simulink model "dbx_control"  (R2015a)
settings: Solver=FixedStepDiscrete  SolverMode=SingleTasking  StartTime=0.0  StopTime=20  FixedStep=T_ctrl  RelTol=1e-3
undefined symbols (not defined in the file): A_l_max_x, A_M, A_z_max, CG, epsilon, Flaps_ang_deg, g, Hover_eta_23, Hover_throtle_1, Hover_throtle_23, I_BAC, L_M, m, Roll_pich_sens, Servo_calib, T_ctrl, Throtle_sens, v_i0, Yaw_sens
libraries: DBX_model x29, DBX_Control_lib x15, simulink x8, DBX_Control x3
(part 2 of 2)

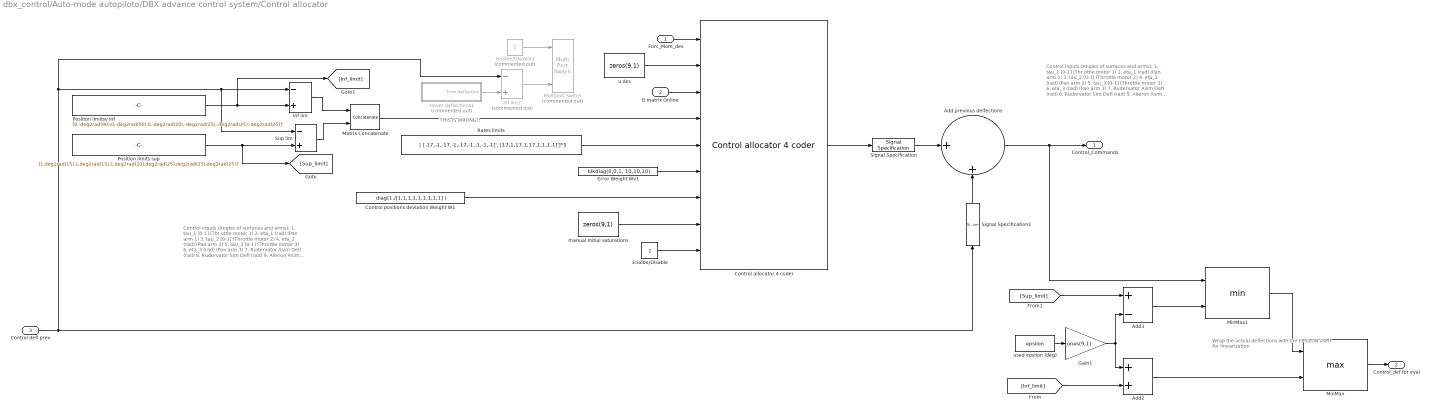
== system dbx_control/Auto-mode autopiloto/DBX advance control system/Control allocator ==
  note: THIS IS WRONG!!
  note: Wrap the actual deflections with the EPSILON
      |  used for linearization
  note: Control inputs (Angles  of surfaces and arms):
      |
      | 1. tau_1 [0-1] (Thr ottle motor 1)
      | 2. eta_1 (rad)  (Pan arm 1)
      |
      | 3. tau_2 [0-1] (Throttle motor 2)
      | 4. eta_2 (rad)  (Pan arm 2)
      |
      | 5. tau_3 [0-1] (Throttle motor 3)
      | 6. eta_3 (rad)  (Pan arm  3)
      |
      | 7. Rudervator Asim Defl (rad)
      | 8. Rudervator Sim Defl (rad)
      | 9. Aileron Asim Defl (rad)
  note: Control inputs (Angles  of surfaces and arms):
      |
      | 1. tau_1 [0-1] (Thr ottle motor 1)
      | 2. eta_1 (rad)  (Pan arm 1)
      |
      | 3. tau_2 [0-1] (Throttle motor 2)
      | 4. eta_2 (rad)  (Pan arm 2)
      |
      | 5. tau_3 [0-1] (Throttle motor 3)
      | 6. eta_3 (rad)  (Pan arm  3)
      |
      | 7. Rudervator Asim Defl (rad)
      | 8. Rudervator Sim Defl (rad)
      | 9. Aileron Asim Defl (rad)
  Forc_Mom_des : Inport
  B matrix Online : Inport  Port=2
  Control defl prev : Inport  Port=3
  Add previous delfections : Sum  Inputs=|++
  Add2 : Sum
  Add3 : Sum  Inputs=+-
  Control allocator 4 coder : DBX_Control_lib/Control allocator 4 coder  gamma=1  imax=20  T=T_ctrl
  Control positions deviation Weight W1 : Constant  Value=diag(1./[1,1,1,1,1,1,1,1,1] )
  Enalbe/Disable : Constant
  Enalbe/Disable1 : Constant  Commented=on
  Error Weight Wv1 : Constant  Value=blkdiag(0,0,1, 10,10,10)
  Gain1 : Gain  Gain=ones(9,1)
  Hover deflections1 : Subsystem  Commented=on  TreatAsAtomicUnit=on
  Inf lim : Sum  Inputs=-+
  Inf lim2 : Sum  Commented=on  Inputs=-+
  Matrix Concatenate : Concatenate  Mode=Multidimensional array  ConcatenateDimension=2
  MinMax : MinMax  Function=max  Inputs=2
  MinMax1 : MinMax  Inputs=2
  Multiport Switch : MultiPortSwitch  Commented=on  Inputs=2
  Position limits sup : Constant  Value=[1,deg2rad(15),1,deg2rad(15),1,deg2rad(20),deg2rad(25),deg2rad(25),deg2rad(25)]'
  Position limitsv inf : Constant  Value=[0,-deg2rad(90),0,-deg2rad(90),0,-deg2rad(20),-deg2rad(25),-deg2rad(25),-deg2rad(25)]'
  Rates limits : Constant  Value=[ [-17,-1,-17,-1,-17,-1,-1,-1,-1]', [17,1,17,1,17,1,1,1,1]']*5
  Signal Specification : SignalSpecification  Dimensions=[9,1]
  Signal Specification1 : SignalSpecification  Dimensions=[9,1]
  Sup lim : Sum  Inputs=-+
  manual Initial saturations : Constant  Value=zeros(9,1)
  u des : Constant  Value=zeros(9,1)
  used epsilon (deg) : Constant  Value=epsilon
  Control_Commands : Outport
  Control_def for eval : Outport  Port=2
  wires:
  MinMax1/1 -> MinMax/1
  Add3/1 -> MinMax1/2
  used epsilon (deg)/1 -> Gain1/1
  Gain1/1 -> Add3/2, Add2/1
  Add2/1 -> MinMax/2
  Control positions deviation Weight W1/1 -> Control allocator 4 coder/7
  Control allocator 4 coder/1 -> Signal Specification/1
  Enalbe/Disable/1 -> Control allocator 4 coder/9
  manual Initial saturations/1 -> Control allocator 4 coder/8
  Sup lim/1 -> Matrix Concatenate/2
  Inf lim/1 -> Matrix Concatenate/1
  Position limitsv inf/1 -> [Inf_limit], Inf lim/2
  Position limits sup/1 -> [Sup_limit], Sup lim/2
  Rates limits/1 -> Control allocator 4 coder/5
  Add previous delfections/1 -> Control_Commands/1, MinMax1/1
  B matrix Online/1 -> Control allocator 4 coder/3
  Signal Specification/1 -> Add previous delfections/1
  Signal Specification1/1 -> Add previous delfections/2
  Forc_Mom_des/1 -> Control allocator 4 coder/1
  Matrix Concatenate/1 -> Control allocator 4 coder/4
  Control defl prev/1 -> Inf lim2/1, Inf lim/1, Sup lim/1, Signal Specification1/1
  Inf lim2/1 -> Multiport Switch/3
  Hover deflections1/1(Trim deflectins) -> Inf lim2/2
  MinMax/1 -> Control_def for eval/1
  Error Weight Wv1/1 -> Control allocator 4 coder/6
  [Inf_limit] -> Add2/2
  [Sup_limit] -> Add3/1
  Enalbe/Disable1/1 -> Multiport Switch/1
  u des/1 -> Control allocator 4 coder/2

== system dbx_control/Auto-mode autopiloto/DBX advance control system/Deflex de-mixer ==
  note: Control outputs:
      |
      | 7. Rudervator Left (rad)
      | 8. Rudervator Right (rad)
      | 9. Aileron Left (rad)
      | 10. Aielron Right (rad)
  delta_rv_Asim : Inport
  delta_rv_sim : Inport  Port=2
  delta_ail_Asim : Inport  Port=3
  delta_ail_sim : Inport  Port=4
  Add : Sum  Inputs=|++
  Add1 : Sum  Inputs=|-+
  Add2 : Sum  Inputs=|++
  Add3 : Sum  Inputs=|-+
  delta_rv_L : Outport
  delta_rv_R : Outport  Port=2
  delta_a_L : Outport  Port=3
  delta_a_R : Outport  Port=4
  wires:
  delta_rv_Asim/1 -> Add1/1, Add/1
  Add/1 -> delta_rv_L/1
  delta_rv_sim/1 -> Add1/2, Add/2
  Add1/1 -> delta_rv_R/1
  delta_ail_Asim/1 -> Add3/1, Add2/1
  Add2/1 -> delta_a_L/1
  delta_ail_sim/1 -> Add2/2, Add3/2
  Add3/1 -> delta_a_R/1

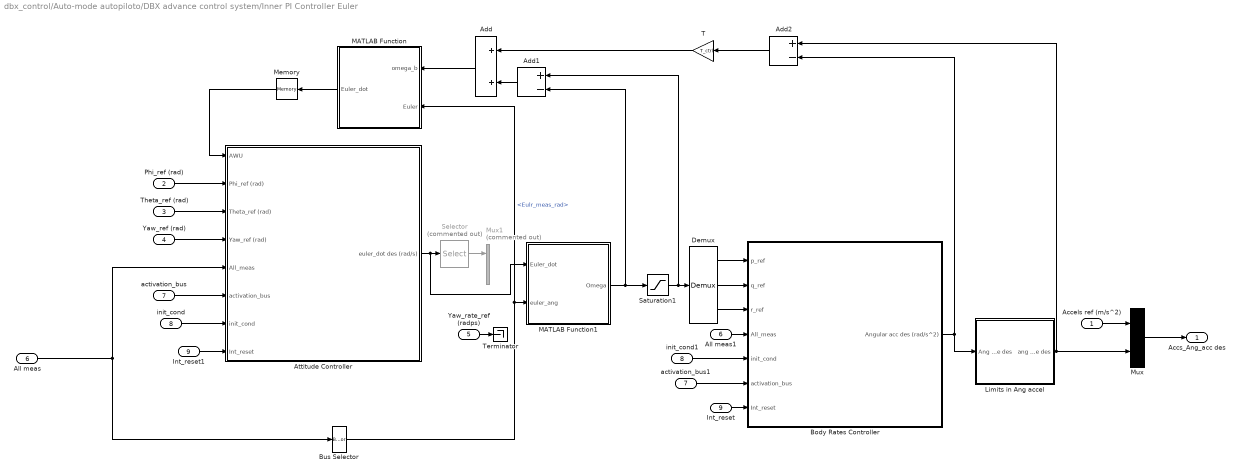
== system dbx_control/Auto-mode autopiloto/DBX advance control system/Inner PI Controller Euler ==
  Accels ref (m/s^2) : Inport
  Phi_ref (rad) : Inport  Port=2
  Theta_ref (rad) : Inport  Port=3
  Yaw_ref (rad) : Inport  Port=4
  Yaw_rate_ref (radps) : Inport  Port=5
  All meas : Inport  Port=6
  activation_bus : Inport  Port=7
  init_cond : Inport  Port=8
  Int_reset : Inport  Port=9
  Add : Sum
  Add1 : Sum  Inputs=+-
  Add2 : Sum  Inputs=+-
  All meas1 : InportShadow  Port=6
  Attitude Controller : Subsystem
  Body Rates Controller : Subsystem
  Bus Selector : BusSelector  OutputSignals=Meas.Eulr_meas_rad
  Demux : Demux  Outputs=3
  Int_reset1 : InportShadow  Port=9
  Limits in Ang accel : Subsystem  TreatAsAtomicUnit=on
  MATLAB Function : MATLAB Function  TreatAsAtomicUnit=on
  MATLAB Function1 : MATLAB Function  TreatAsAtomicUnit=on
  Memory : Memory
  Mux : Mux  Inputs=2
  Mux1 : Mux  Commented=on  Inputs=[2,1]
  Saturation1 : Saturate  UpperLimit=deg2rad(50)*[1,10,0.5]'  LowerLimit=-deg2rad(50)*[1,10,0.5]'
  Selector : Selector  Commented=on  InputPortWidth=3  Indices=[1 2]
  T : Gain  Gain=T_ctrl
  Terminator : Terminator
  activation_bus1 : InportShadow  Port=7
  init_cond1 : InportShadow  Port=8
  Accs_Ang_acc des : Outport
  wires:
  Accels ref (m/s^2)/1 -> Mux/1
  Mux/1 -> Accs_Ang_acc des/1
  All meas/1 -> Bus Selector/1, Attitude Controller/5(All_meas)
  Bus Selector/1 -> MATLAB Function/2(Euler), MATLAB Function1/2(euler_ang)  "<Eulr_meas_rad>"
  Demux/1 -> Body Rates Controller/1(p_ref)
  Demux/2 -> Body Rates Controller/2(q_ref)
  Demux/3 -> Body Rates Controller/3(r_ref)
  Phi_ref (rad)/1 -> Attitude Controller/2(Phi_ref (rad))
  Yaw_ref (rad)/1 -> Attitude Controller/4(Yaw_ref (rad))
  Limits in Ang accel/1(ang Ace des) -> Add2/1, Mux/2
  MATLAB Function1/1(Omega) -> Add1/2, Saturation1/1
  Body Rates Controller/1(Angular acc des (rad/s^2)) -> Add2/2, Limits in Ang accel/1(Ang Ace des)
  Add/1 -> MATLAB Function/1(omega_b)
  Add2/1 -> T/1
  Add1/1 -> Add/2
  T/1 -> Add/1
  MATLAB Function/1(Euler_dot) -> Memory/1
  init_cond/1 -> Attitude Controller/7(init_cond)
  activation_bus/1 -> Attitude Controller/6(activation_bus)
  All meas1/1 -> Body Rates Controller/4(All_meas)
  Saturation1/1 -> Add1/1, Demux/1
  Memory/1 -> Attitude Controller/1(AWU)
  Theta_ref (rad)/1 -> Attitude Controller/3(Theta_ref (rad))
  Selector/1 -> Mux1/1
  Attitude Controller/1(euler_dot des (rad/s)) -> MATLAB Function1/1(Euler_dot), Selector/1
  Int_reset/1 -> Body Rates Controller/7(Int_reset)
  Int_reset1/1 -> Attitude Controller/8(Int_reset)
  activation_bus1/1 -> Body Rates Controller/6(activation_bus)
  init_cond1/1 -> Body Rates Controller/5(init_cond)
  Yaw_rate_ref (radps)/1 -> Terminator/1

== system dbx_control/Auto-mode autopiloto/DBX advance control system/NDI//INDI and Grad4CA ==
  pseudo_control (m/s^2;rad/s^2) : Inport
  Control_defl for eval : Inport  Port=2
  All_meas : Inport  Port=3
  INDI and NDI : Subsystem  RTWFcnName=abc  RTWFileName=asas  VariantControl=NDI_INDI
      settings: RTWFcnNameOpts=User specified  RTWFileNameOpts=User specified
  NDI : Subsystem  RTWFcnName=abc  RTWFileName=asas  VariantControl=NDI
      settings: RTWFcnNameOpts=User specified  RTWFileNameOpts=User specified
  NDI incremental gradient : Subsystem  RTWFcnName=abc  RTWFileName=asas  VariantControl=NDI_incremental_grad
      settings: RTWFcnNameOpts=User specified  RTWFileNameOpts=User specified
  Virtual Control Commands : Outport
  B online : Outport  Port=2
  Control_defl eval (rad) : Outport  Port=3

== system dbx_control/Auto-mode autopiloto/DBX advance control system/Outter Overactuated P Controller ==
  Vel_yaw_ref(m) : Inport
  All meas : Inport  Port=2
  activation_bus : Inport  Port=3
  init_cond : Inport  Port=4
  Int_reset : Inport  Port=5
  Bus Selector1 : BusSelector  OutputSignals=Params.T_Fe_Fyaw,Meas.V_yaw,Params.DCM
  Demux2 : Demux  Outputs=3
  Matrix Multiply1 : Product  Multiplication=Matrix(*)
  Matrix Multiply3 : Product  Multiplication=Matrix(*)
  Permute Dimensions : PermuteDimensions
  Permute Dimensions1 : PermuteDimensions
  Saturation : Saturate  UpperLimit=[A_l_max_x,10,g]  LowerLimit=-[A_l_max_x,10,A_z_max-g]
  Saturation1 : Saturate  UpperLimit=[10,10,v_i0]'  LowerLimit=-[10,10,2*v_i0]'
  Terminator : Terminator
  Velocity Controller : Subsystem
  Accels des : Outport
  wires:
  Demux2/3 -> Velocity Controller/2(Vyaw_z_ref)
  Demux2/1 -> Velocity Controller/1(Vyaw_x_ref)
  All meas/1 -> Bus Selector1/1
  Bus Selector1/3 -> Permute Dimensions/1  "<DCM>"
  Matrix Multiply1/1 -> Accels des/1
  Permute Dimensions/1 -> Matrix Multiply1/1
  Saturation1/1 -> Demux2/1
  Saturation/1 -> Matrix Multiply3/2
  Bus Selector1/1 -> Permute Dimensions1/1  "<T_Fe_Fyaw>"
  Vel_yaw_ref(m)/1 -> Saturation1/1
  Matrix Multiply3/1 -> Matrix Multiply1/2  "in F_e"
  Permute Dimensions1/1 -> Matrix Multiply3/1
  Velocity Controller/1(Acc_yaw des (m/s)) -> Saturation/1
  activation_bus/1 -> Velocity Controller/4(activation_bus)
  Bus Selector1/2 -> Velocity Controller/3(V_yaw_meas)  "<V_yaw>"
  init_cond/1 -> Velocity Controller/5(Init_cond)
  Demux2/2 -> Terminator/1
  Int_reset/1 -> Velocity Controller/6(Int_reset)

== system dbx_control/Auto-mode autopiloto/DBX advance control system/keep -90//90 ==
  in (rad) : Inport
  Constant : Constant  Value=180
  Constant2 : Constant  Value=360
  Gain : Gain  Gain=360
  Math Function2 : Math  Operator=rem  SaturateOnIntegerOverflow=on
  Product : Product  Inputs=*/  RndMeth=Zero
  Rounding Function : Rounding  Operator=fix
  Sum2 : Sum  Inputs=|-+
  deg2rad1 : Gain  Gain=pi/180  SaturateOnIntegerOverflow=on  OutDataTypeStr=Inherit: Same as input  ParamDataTypeStr=Inherit: Same as input
  rad2deg : Gain  Gain=180/pi  SaturateOnIntegerOverflow=on  OutDataTypeStr=Inherit: Same as input  ParamDataTypeStr=Inherit: Same as input
  out (rad) : Outport
  wires:
  deg2rad1/1 -> out (rad)/1
  Sum2/1 -> deg2rad1/1
  Math Function2/1 -> Sum2/2, Product/1
  Constant2/1 -> Math Function2/2
  rad2deg/1 -> Math Function2/1
  Gain/1 -> Sum2/1
  Rounding Function/1 -> Gain/1
  Product/1 -> Rounding Function/1
  Constant/1 -> Product/2
  in (rad)/1 -> rad2deg/1

== system dbx_control/Auto-mode autopiloto/DBX advance control system/Control allocator/Hover deflections1 ==
  Contro Inputs1 : Constant  Value=Hover_throtle_1
  Contro Inputs2 : Constant  Value=Hover_throtle_23
  Contro Inputs3 : Constant  Value=Hover_eta_23
  Gain : Gain  Gain=-1
  Ground : Ground
  Mux : Mux  Inputs=9
  Trim deflectins : Outport
  wires:
  Contro Inputs1/1 -> Mux/1
  Contro Inputs2/1 -> Mux/7, Mux/4
  Ground/1 -> Mux/2, Mux/6, Mux/9, Mux/3
  Contro Inputs3/1 -> Gain/1, Mux/5
  Gain/1 -> Mux/8
  Mux/1 -> Trim deflectins/1

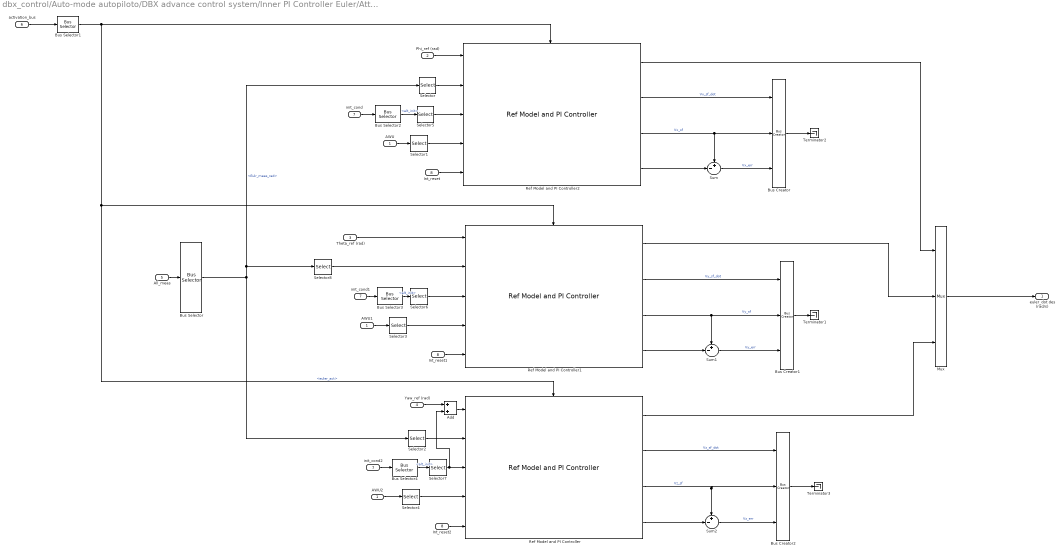
== system dbx_control/Auto-mode autopiloto/DBX advance control system/Inner PI Controller Euler/Attitude Controller ==
  AWU : Inport
  Phi_ref (rad) : Inport  Port=2
  Theta_ref (rad) : Inport  Port=3
  Yaw_ref (rad) : Inport  Port=4
  All_meas : Inport  Port=5
  activation_bus : Inport  Port=6
  init_cond : Inport  Port=7
  Int_reset : Inport  Port=8
  AWU1 : InportShadow
  AWU2 : InportShadow
  Add : Sum
  Bus Creator : BusCreator  Inputs=3
  Bus Creator1 : BusCreator  Inputs=3
  Bus Creator2 : BusCreator  Inputs=3
  Bus Selector : BusSelector  OutputSignals=Meas.Eulr_meas_rad
  Bus Selector1 : BusSelector  OutputSignals=euler_act
  Bus Selector2 : BusSelector  OutputSignals=alt_init
  Bus Selector3 : BusSelector  OutputSignals=alt_init
  Bus Selector4 : BusSelector  OutputSignals=alt_init
  Int_reset1 : InportShadow  Port=8
  Int_reset2 : InportShadow  Port=8
  Mux : Mux  Inputs=3
  Ref Model and PI Controller : DBX_Control_lib/Ref Model and PI Controller  delta=0  tau=psi_tau  RisingSlewLimit=deg2rad(20)  FallingSlewLimit=-deg2rad(20)  K_f=0  K_a=1  Con_way=pro  omega_n=4  xi=0.5  Z1=-30  K_b=psi_K_b  f_i=psi_f_i  f_c=1
  Ref Model and PI Controller1 : DBX_Control_lib/Ref Model and PI Controller  delta=0  tau=theta_tau  RisingSlewLimit=deg2rad(20)  FallingSlewLimit=-deg2rad(20)  K_f=0  K_a=1  Con_way=pro  omega_n=4  xi=0.5  Z1=-30  K_b=theta_K_b  f_i=theta_f_i  f_c=1
  Ref Model and PI Controller2 : DBX_Control_lib/Ref Model and PI Controller  delta=0  tau=phi_tau  RisingSlewLimit=deg2rad(20)  FallingSlewLimit=-deg2rad(20)  K_f=0  K_a=1  Con_way=pro  omega_n=4  xi=0.5  Z1=-30  K_b=phi_K_b  f_i=phi_f_i  f_c=1
  Selector : Selector  InputPortWidth=3
  Selector1 : Selector  InputPortWidth=3
  Selector2 : Selector  InputPortWidth=3  Indices=3
  Selector3 : Selector  InputPortWidth=3  Indices=2
  Selector4 : Selector  InputPortWidth=3  Indices=3
  Selector5 : Selector  InputPortWidth=3
  Selector6 : Selector  InputPortWidth=3  Indices=2
  Selector7 : Selector  InputPortWidth=3  Indices=3
  Selector8 : Selector  InputPortWidth=3  Indices=2
  Sum : Sum  Inputs=+-|
  Sum1 : Sum  Inputs=+-|
  Sum2 : Sum  Inputs=+-|
  Terminator1 : Terminator
  Terminator2 : Terminator
  Terminator3 : Terminator
  init_cond1 : InportShadow  Port=7
  init_cond2 : InportShadow  Port=7
  euler_dot des (rad/s) : Outport
  wires:
  Ref Model and PI Controller/4 -> Sum2/2
  Sum2/1 -> Bus Creator2/3  "Vz_err"
  Ref Model and PI Controller/3 -> Bus Creator2/2, Sum2/1  "Vz_sf"
  Ref Model and PI Controller/2 -> Bus Creator2/1  "Vz_sf_dot"
  Ref Model and PI Controller1/4 -> Sum1/2
  Sum1/1 -> Bus Creator1/3  "Vy_err"
  Ref Model and PI Controller1/3 -> Sum1/1, Bus Creator1/2  "Vy_sf"
  Ref Model and PI Controller1/2 -> Bus Creator1/1  "Vy_sf_dot"
  Ref Model and PI Controller2/4 -> Sum/2
  Bus Creator2/1 -> Terminator3/1
  Bus Creator1/1 -> Terminator1/1
  Bus Creator/1 -> Terminator2/1
  Sum/1 -> Bus Creator/3  "Vx_err"
  Ref Model and PI Controller2/3 -> Sum/1, Bus Creator/2  "Vx_sf"
  Ref Model and PI Controller2/2 -> Bus Creator/1  "Vx_sf_dot"
  Yaw_ref (rad)/1 -> Add/1
  Selector/1 -> Ref Model and PI Controller2/2
  All_meas/1 -> Bus Selector/1
  Phi_ref (rad)/1 -> Ref Model and PI Controller2/1
  Mux/1 -> euler_dot des (rad/s)/1
  Ref Model and PI Controller2/1 -> Mux/1
  Ref Model and PI Controller/1 -> Mux/3
  Ref Model and PI Controller1/1 -> Mux/2
  Selector2/1 -> Ref Model and PI Controller/2
  Bus Selector/1 -> Selector/1, Selector8/1, Selector2/1  "<Eulr_meas_rad>"
  Selector8/1 -> Ref Model and PI Controller1/2
  Theta_ref (rad)/1 -> Ref Model and PI Controller1/1
  AWU/1 -> Selector1/1
  AWU1/1 -> Selector3/1
  AWU2/1 -> Selector4/1
  Selector1/1 -> Ref Model and PI Controller2/4
  Selector3/1 -> Ref Model and PI Controller1/4
  Selector4/1 -> Ref Model and PI Controller/4
  activation_bus/1 -> Bus Selector1/1
  Bus Selector1/1 -> Ref Model and PI Controller/Enable, Ref Model and PI Controller1/Enable, Ref Model and PI Controller2/Enable  "<euler_act>"
  init_cond/1 -> Bus Selector2/1
  Bus Selector2/1 -> Selector5/1  "<alt_init>"
  Selector5/1 -> Ref Model and PI Controller2/3
  Selector6/1 -> Ref Model and PI Controller1/3
  init_cond1/1 -> Bus Selector3/1
  Bus Selector3/1 -> Selector6/1  "<alt_init>"
  init_cond2/1 -> Bus Selector4/1
  Selector7/1 -> Add/2, Ref Model and PI Controller/3
  Bus Selector4/1 -> Selector7/1  "<alt_init>"
  Int_reset/1 -> Ref Model and PI Controller2/5
  Int_reset1/1 -> Ref Model and PI Controller1/5
  Int_reset2/1 -> Ref Model and PI Controller/5
  Add/1 -> Ref Model and PI Controller/1

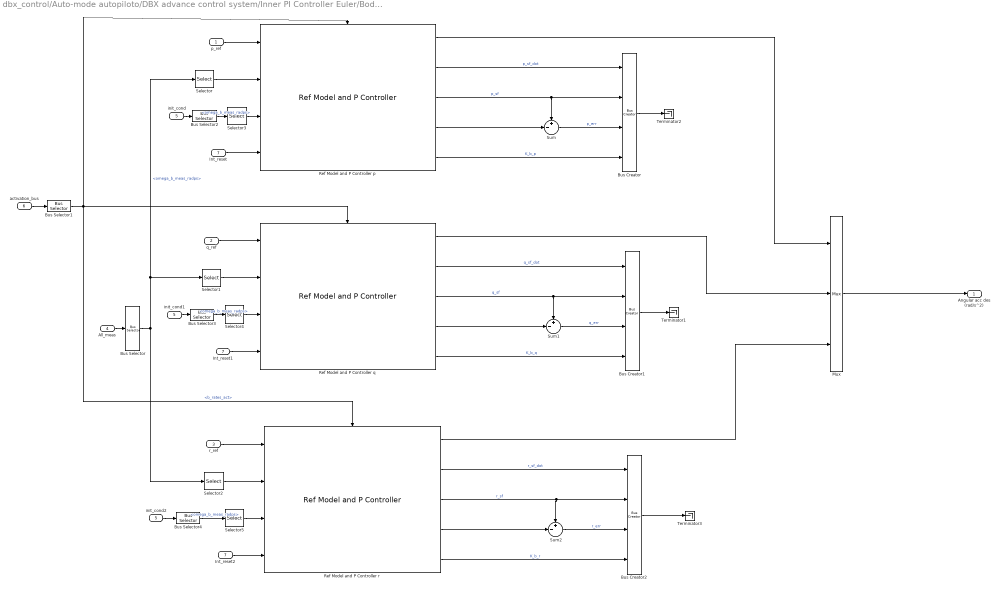
== system dbx_control/Auto-mode autopiloto/DBX advance control system/Inner PI Controller Euler/Body Rates Controller ==
  p_ref : Inport
  q_ref : Inport  Port=2
  r_ref : Inport  Port=3
  All_meas : Inport  Port=4
  init_cond : Inport  Port=5
  activation_bus : Inport  Port=6
  Int_reset : Inport  Port=7
  Bus Creator : BusCreator
  Bus Creator1 : BusCreator
  Bus Creator2 : BusCreator
  Bus Selector : BusSelector  OutputSignals=Meas.omega_b_meas_radps
  Bus Selector1 : BusSelector  OutputSignals=b_rates_act
  Bus Selector2 : BusSelector  OutputSignals=omega_b_meas_radps
  Bus Selector3 : BusSelector  OutputSignals=omega_b_meas_radps
  Bus Selector4 : BusSelector  OutputSignals=omega_b_meas_radps
  Int_reset1 : InportShadow  Port=7
  Int_reset2 : InportShadow  Port=7
  Mux : Mux  Inputs=3
  Ref Model and P Controller p : DBX_Control_lib/Ref Model and P Controller  tau=p_tau  RisingSlewLimit=4  FallingSlewLimit=-4  K_f=0.5  K_b=p_K_b
  Ref Model and P Controller q : DBX_Control_lib/Ref Model and P Controller  tau=q_tau  RisingSlewLimit=4  FallingSlewLimit=-4  K_f=0.5  K_b=q_K_b
  Ref Model and P Controller r : DBX_Control_lib/Ref Model and P Controller  tau=r_tau  RisingSlewLimit=4  FallingSlewLimit=-4  K_f=0.1  K_b=r_K_b
  Selector : Selector  InputPortWidth=3
  Selector1 : Selector  InputPortWidth=3  Indices=2
  Selector2 : Selector  InputPortWidth=3  Indices=3
  Selector3 : Selector  InputPortWidth=3
  Selector4 : Selector  InputPortWidth=3  Indices=2
  Selector5 : Selector  InputPortWidth=3  Indices=[3]
  Sum : Sum  Inputs=+-|
  Sum1 : Sum  Inputs=+-|
  Sum2 : Sum  Inputs=+-|
  Terminator1 : Terminator
  Terminator2 : Terminator
  Terminator3 : Terminator
  init_cond1 : InportShadow  Port=5
  init_cond2 : InportShadow  Port=5
  Angular acc des (rad/s^2) : Outport
  wires:
  Ref Model and P Controller r/5 -> Bus Creator2/4  "K_b_r"
  Ref Model and P Controller r/4 -> Sum2/2
  Sum2/1 -> Bus Creator2/3  "r_err"
  Ref Model and P Controller r/3 -> Bus Creator2/2, Sum2/1  "r_sf"
  Ref Model and P Controller r/2 -> Bus Creator2/1  "r_sf_dot"
  Ref Model and P Controller q/5 -> Bus Creator1/4  "K_b_q"
  Ref Model and P Controller q/4 -> Sum1/2
  Sum1/1 -> Bus Creator1/3  "q_err"
  Ref Model and P Controller q/3 -> Bus Creator1/2, Sum1/1  "q_sf"
  Ref Model and P Controller q/2 -> Bus Creator1/1  "q_sf_dot"
  Ref Model and P Controller p/5 -> Bus Creator/4  "K_b_p"
  Ref Model and P Controller p/4 -> Sum/2
  Selector2/1 -> Ref Model and P Controller r/2
  Bus Creator2/1 -> Terminator3/1
  Bus Creator1/1 -> Terminator1/1
  Bus Creator/1 -> Terminator2/1
  Sum/1 -> Bus Creator/3  "p_err"
  Ref Model and P Controller p/3 -> Bus Creator/2, Sum/1  "p_sf"
  Ref Model and P Controller p/2 -> Bus Creator/1  "p_sf_dot"
  r_ref/1 -> Ref Model and P Controller r/1
  Selector1/1 -> Ref Model and P Controller q/2
  q_ref/1 -> Ref Model and P Controller q/1
  Mux/1 -> Angular acc des (rad/s^2)/1
  p_ref/1 -> Ref Model and P Controller p/1
  Bus Selector/1 -> Selector2/1, Selector/1, Selector1/1  "<omega_b_meas_radps>"
  All_meas/1 -> Bus Selector/1
  Ref Model and P Controller r/1 -> Mux/3
  Ref Model and P Controller q/1 -> Mux/2
  Ref Model and P Controller p/1 -> Mux/1
  Selector/1 -> Ref Model and P Controller p/2
  activation_bus/1 -> Bus Selector1/1
  Bus Selector1/1 -> Ref Model and P Controller p/Enable, Ref Model and P Controller r/Enable, Ref Model and P Controller q/Enable  "<b_rates_act>"
  init_cond/1 -> Bus Selector2/1
  Bus Selector2/1 -> Selector3/1  "<omega_b_meas_radps>"
  Selector3/1 -> Ref Model and P Controller p/3
  init_cond1/1 -> Bus Selector3/1
  Bus Selector3/1 -> Selector4/1  "<omega_b_meas_radps>"
  Selector4/1 -> Ref Model and P Controller q/3
  init_cond2/1 -> Bus Selector4/1
  Bus Selector4/1 -> Selector5/1  "<omega_b_meas_radps>"
  Selector5/1 -> Ref Model and P Controller r/3
  Int_reset/1 -> Ref Model and P Controller p/4
  Int_reset1/1 -> Ref Model and P Controller q/4
  Int_reset2/1 -> Ref Model and P Controller r/4

== system dbx_control/Auto-mode autopiloto/DBX advance control system/Inner PI Controller Euler/Limits in Ang accel ==
  note: Here it is assumed that at all time every prop is generating m*g/3 newtons of force . It is conservative?
  Ang Ace des : Inport
  Limis eval : MATLAB Function  TreatAsAtomicUnit=on
  Saturation Dynamic : simulink/Discontinuities/Saturation Dynamic  OutMin=[]  OutMax=[]  OutDataTypeStr=Inherit: Same as second input  OutDataType=fixdt(1, 16)  OutScaling=2^-10  DoSatur=off
  ang Ace des : Outport
  wires:
  Limis eval/1(Limit_up) -> Saturation Dynamic/1
  Limis eval/2(Limit_down) -> Saturation Dynamic/3
  Ang Ace des/1 -> Saturation Dynamic/2, Limis eval/1(Ang_Accel)
  Saturation Dynamic/1 -> ang Ace des/1

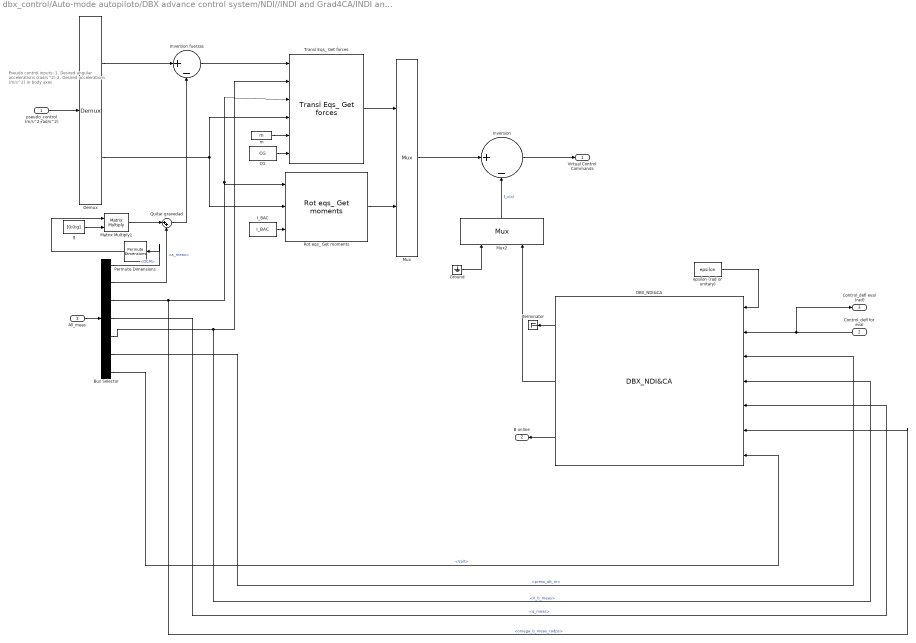
== system dbx_control/Auto-mode autopiloto/DBX advance control system/NDI//INDI and Grad4CA/INDI and NDI ==
  note: Pseudo control inputs:
      | 1. Desired angular accelerations (rad/s^2)
      | 2. Desired accelerations (m/s^2) in body axes
  pseudo_control (m/s^2;rad/s^2) : Inport
  Control_defl for eval : Inport  Port=2
  All_meas : Inport  Port=3
  Bus Selector : BusSelector  OutputSignals=Params.DCM,Meas.a_meas,Meas.omega_b_meas_radps,Meas.q_meas,Meas.V_b_meas,Meas.press_alt_m,Meas.Volt
  CG : Constant  Value=CG
  DBX_NDI&CA : DBX_Control/DBX_NDI&CA  SystemSampleTime=-1
  Demux : Demux  Outputs=[3,3]
  Ground : Ground
  I_BAC : Constant  Value=I_BAC
  Inversion : Sum  Inputs=|+-
  Inversion fuerzas : Sum  Inputs=|+-
  Matrix Multiply1 : Product  Multiplication=Matrix(*)
  Mux : Mux  Inputs=[3,3]
  Mux2 : Mux  Inputs=[3,3]
  Permute Dimensions : PermuteDimensions
  Quitar gravedad : Sum  Inputs=|++
  Rot eqs_ Get moments : DBX_Control/Rot eqs_ Get moments
  Terminator : Terminator
  Transl Eqs_ Get forces : DBX_Control/Transl Eqs_ Get forces
  epsilon (rad or unitary) : Constant  Value=epsilon
  g : Constant  Value=[0;0;g]
  m : Constant  Value=m
  Virtual Control Commands : Outport
  B online : Outport  Port=2
  Control_defl eval (rad) : Outport  Port=3
  wires:
  DBX_NDI&CA/3 -> B online/1
  Mux/1 -> Inversion/1
  Mux2/1 -> Inversion/2  "f_x(x)"
  All_meas/1 -> Bus Selector/1
  pseudo_control (m/s^2;rad/s^2)/1 -> Demux/1
  Demux/2 -> Rot eqs_ Get moments/2, Transl Eqs_ Get forces/4
  Demux/1 -> Inversion fuerzas/1
  Bus Selector/3 -> Transl Eqs_ Get forces/3, Rot eqs_ Get moments/1, DBX_NDI&CA/6  "<omega_b_meas_radps>"
  Bus Selector/5 -> DBX_NDI&CA/4, Transl Eqs_ Get forces/2  "<V_b_meas>"
  Control_defl for eval/1 -> DBX_NDI&CA/2, Control_defl eval (rad)/1
  Bus Selector/6 -> DBX_NDI&CA/3  "<press_alt_m>"
  Bus Selector/4 -> DBX_NDI&CA/5  "<q_meas>"
  m/1 -> Transl Eqs_ Get forces/5
  epsilon (rad or unitary)/1 -> DBX_NDI&CA/1
  Transl Eqs_ Get forces/1 -> Mux/1
  Rot eqs_ Get moments/1 -> Mux/2
  DBX_NDI&CA/2 -> Mux2/2
  Inversion/1 -> Virtual Control Commands/1
  Bus Selector/7 -> DBX_NDI&CA/7  "<Volt>"
  I_BAC/1 -> Rot eqs_ Get moments/3
  CG/1 -> Transl Eqs_ Get forces/6
  Ground/1 -> Mux2/1
  Inversion fuerzas/1 -> Transl Eqs_ Get forces/1
  DBX_NDI&CA/1 -> Terminator/1
  Permute Dimensions/1 -> Matrix Multiply1/1
  g/1 -> Matrix Multiply1/2
  Bus Selector/2 -> Quitar gravedad/2  "<a_meas>"
  Quitar gravedad/1 -> Inversion fuerzas/2
  Matrix Multiply1/1 -> Quitar gravedad/1
  Bus Selector/1 -> Permute Dimensions/1  "<DCM>"

== system dbx_control/Auto-mode autopiloto/DBX advance control system/NDI//INDI and Grad4CA/NDI ==
  note: Pseudo control inputs:
      | 1. Desired angular accelerations (rad/s^2)
      | 2. Desired accelerations (m/s^2) in body axes
  pseudo_control (m/s^2;rad/s^2) : Inport
  Control_defl for eval : Inport  Port=2
  All_meas : Inport  Port=3
  Bus Selector : BusSelector  OutputSignals=Meas.omega_b_meas_radps,Meas.q_meas,Meas.V_b_meas,Meas.press_alt_m,Meas.Volt
  CG : Constant  Value=CG
  DBX_NDI&CA : DBX_Control_lib/DBX_NDI&CA  SystemSampleTime=-1
  Demux : Demux  Outputs=[3,3]
  I_BAC : Constant  Value=I_BAC
  Inversion : Sum  Inputs=|+-
  Mux : Mux  Inputs=[3,3]
  Mux2 : Mux  Inputs=[3,3]
  Rot eqs_ Get moments : DBX_Control_lib/Rot eqs_ Get moments
  Transl Eqs_ Get forces : DBX_Control_lib/Transl Eqs_ Get forces
  epsilon (rad or unitary) : Constant  Value=epsilon
  m : Constant  Value=m
  Virtual Control Commands : Outport
  B online : Outport  Port=2
  Control_defl eval (rad) : Outport  Port=3
  wires:
  CG/1 -> Transl Eqs_ Get forces/6
  I_BAC/1 -> Rot eqs_ Get moments/3
  Bus Selector/5 -> DBX_NDI&CA/7  "<Volt>"
  Inversion/1 -> Virtual Control Commands/1
  DBX_NDI&CA/2 -> Mux2/2
  DBX_NDI&CA/1 -> Mux2/1
  Rot eqs_ Get moments/1 -> Mux/2
  Transl Eqs_ Get forces/1 -> Mux/1
  epsilon (rad or unitary)/1 -> DBX_NDI&CA/1
  m/1 -> Transl Eqs_ Get forces/5
  Bus Selector/2 -> DBX_NDI&CA/5  "<q_meas>"
  Bus Selector/4 -> DBX_NDI&CA/3  "<press_alt_m>"
  Control_defl for eval/1 -> Control_defl eval (rad)/1, DBX_NDI&CA/2
  Bus Selector/3 -> Transl Eqs_ Get forces/2, DBX_NDI&CA/4  "<V_b_meas>"
  Bus Selector/1 -> Rot eqs_ Get moments/1, Transl Eqs_ Get forces/3, DBX_NDI&CA/6  "<omega_b_meas_radps>"
  Demux/1 -> Transl Eqs_ Get forces/1
  Demux/2 -> Transl Eqs_ Get forces/4, Rot eqs_ Get moments/2
  pseudo_control (m/s^2;rad/s^2)/1 -> Demux/1
  All_meas/1 -> Bus Selector/1
  Mux2/1 -> Inversion/2  "f_x(x)"
  Mux/1 -> Inversion/1
  DBX_NDI&CA/3 -> B online/1

== system dbx_control/Auto-mode autopiloto/DBX advance control system/NDI//INDI and Grad4CA/NDI incremental gradient ==
  note: Pseudo control inputs:
      | 1. Desired angular accelerations (rad/s^2)
      | 2. Desired accelerations (m/s^2) in body axes
  pseudo_control (m/s^2;rad/s^2) : Inport
  Control_defl for eval : Inport  Port=2
  All_meas : Inport  Port=3
  Bus Selector : BusSelector  OutputSignals=Meas.omega_b_meas_radps,Meas.q_meas,Meas.V_b_meas,Meas.press_alt_m,Meas.Volt
  CG : Constant  Value=CG
  DBX_NDI&CA Incremental Gradient : DBX_Control_lib/DBX_NDI&CA Incremental Gradient  SystemSampleTime=-1
  Demux : Demux  Outputs=[3,3]
  I_BAC : Constant  Value=I_BAC
  Inversion : Sum  Inputs=|+-
  Mux : Mux  Inputs=[3,3]
  Mux2 : Mux  Inputs=[3,3]
  Rot eqs_ Get moments : DBX_Control_lib/Rot eqs_ Get moments
  Transl Eqs_ Get forces : DBX_Control_lib/Transl Eqs_ Get forces
  epsilon (rad or unitary) : Constant  Value=epsilon
  m : Constant  Value=m
  Virtual Control Commands : Outport
  B online : Outport  Port=2
  Control_defl eval (rad) : Outport  Port=3
  wires:
  DBX_NDI&CA Incremental Gradient/3 -> B online/1
  Mux/1 -> Inversion/1
  Mux2/1 -> Inversion/2  "f_x(x)"
  All_meas/1 -> Bus Selector/1
  pseudo_control (m/s^2;rad/s^2)/1 -> Demux/1
  Demux/2 -> Rot eqs_ Get moments/2, Transl Eqs_ Get forces/4
  Demux/1 -> Transl Eqs_ Get forces/1
  Bus Selector/1 -> DBX_NDI&CA Incremental Gradient/6, Transl Eqs_ Get forces/3, Rot eqs_ Get moments/1  "<omega_b_meas_radps>"
  Bus Selector/3 -> DBX_NDI&CA Incremental Gradient/4, Transl Eqs_ Get forces/2  "<V_b_meas>"
  Control_defl for eval/1 -> DBX_NDI&CA Incremental Gradient/2, Control_defl eval (rad)/1
  Bus Selector/4 -> DBX_NDI&CA Incremental Gradient/3  "<press_alt_m>"
  Bus Selector/2 -> DBX_NDI&CA Incremental Gradient/5  "<q_meas>"
  m/1 -> Transl Eqs_ Get forces/5
  epsilon (rad or unitary)/1 -> DBX_NDI&CA Incremental Gradient/1
  Transl Eqs_ Get forces/1 -> Mux/1
  Rot eqs_ Get moments/1 -> Mux/2
  DBX_NDI&CA Incremental Gradient/1 -> Mux2/1
  DBX_NDI&CA Incremental Gradient/2 -> Mux2/2
  Inversion/1 -> Virtual Control Commands/1
  Bus Selector/5 -> DBX_NDI&CA Incremental Gradient/7  "<Volt>"
  I_BAC/1 -> Rot eqs_ Get moments/3
  CG/1 -> Transl Eqs_ Get forces/6

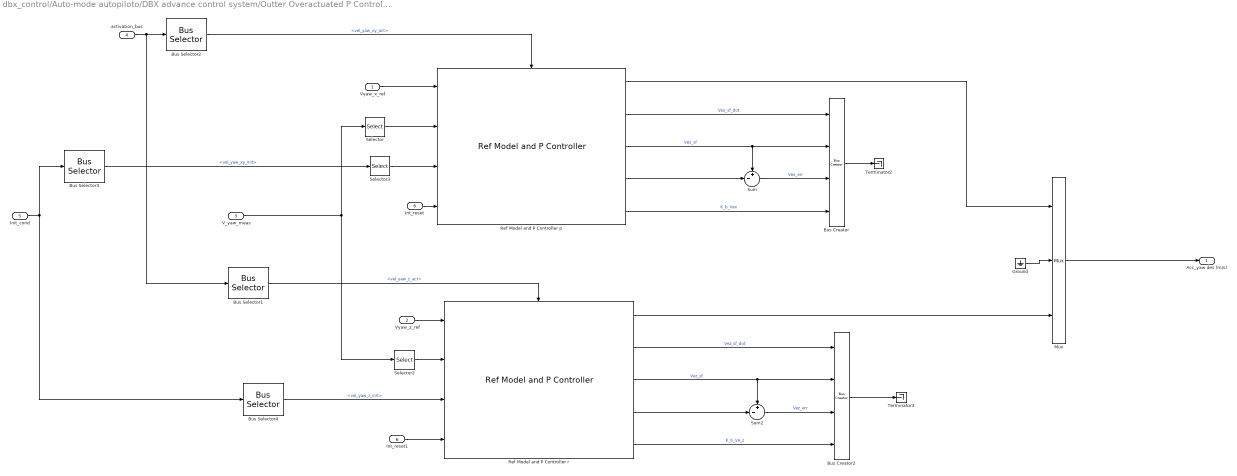
== system dbx_control/Auto-mode autopiloto/DBX advance control system/Outter Overactuated P Controller/Velocity Controller ==
  Vyaw_x_ref : Inport
  Vyaw_z_ref : Inport  Port=2
  V_yaw_meas : Inport  Port=3
  activation_bus : Inport  Port=4
  Init_cond : Inport  Port=5
  Int_reset : Inport  Port=6
  Bus Creator : BusCreator
  Bus Creator2 : BusCreator
  Bus Selector1 : BusSelector  OutputSignals=vel_yaw_z_act
  Bus Selector2 : BusSelector  OutputSignals=vel_yaw_xy_act
  Bus Selector3 : BusSelector  OutputSignals=vel_yaw_xy_init
  Bus Selector4 : BusSelector  OutputSignals=vel_yaw_z_init
  Ground : Ground
  Int_reset1 : InportShadow  Port=6
  Mux : Mux  Inputs=3
  Ref Model and P Controller p : DBX_Control_lib/Ref Model and P Controller  tau=2  RisingSlewLimit=1  FallingSlewLimit=-1  K_f=0.5  K_b=1
  Ref Model and P Controller r : DBX_Control_lib/Ref Model and P Controller  tau=1  RisingSlewLimit=1  FallingSlewLimit=-1  K_f=0.4  K_b=8
  Selector : Selector  InputPortWidth=3
  Selector2 : Selector  InputPortWidth=3  Indices=3
  Selector3 : Selector  InputPortWidth=2
  Sum : Sum  Inputs=+-|
  Sum2 : Sum  Inputs=+-|
  Terminator2 : Terminator
  Terminator3 : Terminator
  Acc_yaw des (m/s) : Outport
  wires:
  Ref Model and P Controller r/5 -> Bus Creator2/4  "K_b_Ve_z"
  Ref Model and P Controller r/4 -> Sum2/2
  Sum2/1 -> Bus Creator2/3  "Vez_err"
  Ref Model and P Controller r/3 -> Bus Creator2/2, Sum2/1  "Vez_sf"
  Ref Model and P Controller r/2 -> Bus Creator2/1  "Vez_sf_dot"
  Ref Model and P Controller p/5 -> Bus Creator/4  "K_b_Vex"
  Ref Model and P Controller p/4 -> Sum/2
  Selector2/1 -> Ref Model and P Controller r/2
  Bus Creator2/1 -> Terminator3/1
  Bus Creator/1 -> Terminator2/1
  Sum/1 -> Bus Creator/3  "Vex_err"
  Ref Model and P Controller p/3 -> Bus Creator/2, Sum/1  "Vex_sf"
  Ref Model and P Controller p/2 -> Bus Creator/1  "Vex_sf_dot"
  Ref Model and P Controller r/1 -> Mux/3
  Vyaw_z_ref/1 -> Ref Model and P Controller r/1
  Mux/1 -> Acc_yaw des (m/s)/1
  Ref Model and P Controller p/1 -> Mux/1
  Vyaw_x_ref/1 -> Ref Model and P Controller p/1
  V_yaw_meas/1 -> Selector/1, Selector2/1
  Selector/1 -> Ref Model and P Controller p/2
  activation_bus/1 -> Bus Selector1/1, Bus Selector2/1
  Bus Selector2/1 -> Ref Model and P Controller p/Enable  "<vel_yaw_xy_act>"
  Bus Selector1/1 -> Ref Model and P Controller r/Enable  "<vel_yaw_z_act>"
  Init_cond/1 -> Bus Selector4/1, Bus Selector3/1
  Bus Selector3/1 -> Selector3/1  "<vel_yaw_xy_init>"
  Selector3/1 -> Ref Model and P Controller p/3
  Bus Selector4/1 -> Ref Model and P Controller r/3  "<vel_yaw_z_init>"
  Ground/1 -> Mux/2
  Int_reset1/1 -> Ref Model and P Controller r/4
  Int_reset/1 -> Ref Model and P Controller p/4

== matlab function dbx_control/Manual flight mode/pwm_out1 ==
  data: Roll input; M1 output size=1; P input size=1; Y input size=1; T input size=1; M2 output size=1; M3 output size=1; S3 output size=1; R parameter
function [M1, M2, M3, S3] = motor_mixer(Roll, P, Y, T,R)
%% Salidas de Throtle de -1 a 1 y angulos en rad
idle_motor = 0;

% DBX

M1 = max(T+Roll/2+P/3,0);
M2 = max(T-Roll/2+P/3,0);
M3 = max(T-2*P/3,0);


S3 = 0.3*R/(max(T-2*P/3,0.2))*(T-Y) ;

% Quad X
% M1 = ((Roll + Pitch - Yaw) / 2 * Thrust + Thrust) * 1000 + idle_motor;
% M2 = ((-Roll + Pitch + Yaw) / 2 * Thrust + Thrust) * 1000 + idle_motor;
% M3 = ((-Roll - Pitch - Yaw) / 2 * Thrust + Thrust) * 1000 + idle_motor;
% S3 = ((Roll - Pitch + Yaw) / 2 * Thrust + Thrust) * 1000 + idle_motor;
% M5 = 1000;
% M6 = 1000;
% M7 = 1000;
% M8 = 1000;

% Quad +
% M1 = ((Pitch - Yaw) * Thrust / 2 + Thrust) * 1000 + idle_PWM;
% M2 = ((-Roll + Yaw) * Thrust / 2 + Thrust) * 1000 + idle_PWM;
% M3 = ((-Pitch - Yaw) * Thrust / 2 + Thrust) * 1000 + idle_PWM;
% M4 = ((Roll + Yaw) * Thrust / 2 + Thrust) * 1000 + idle_PWM;
% M5 = 1000;
% M6 = 1000;
% M7 = 1000;
% M8 = 1000;

% Hex X
% M1 = ((Pitch + Roll / 2 - Yaw) * Thrust / 2 + Thrust) * 1000 + idle_PWM;
% M2 = ((Pitch - Roll / 2 + Yaw) * Thrust / 2 + Thrust) * 1000 + idle_PWM;
% M3 = ((-Roll - Yaw) * Thrust / 2 + Thrust) * 1000 + idle_PWM;
% M4 = ((-Pitch - Roll / 2 + Yaw) * Thrust / 2 + Thrust) * 1000 + idle_PWM;
% M5 = ((-Pitch + Roll / 2 - Yaw) * Thrust / 2 + Thrust) * 1000 + idle_PWM;
% M6 = ((Roll + Yaw) * Thrust / 2 + Thrust) * 1000 + idle_PWM;
% M7 = 1000;
% M8 = 1000;


end

== matlab function dbx_control/Auto-mode autopiloto/DBX advance control system/Inner PI Controller Euler/MATLAB Function ==
  data: omega_b input size=[3,1]; Euler_dot output; Euler input size=[3,1]
function Euler_dot = omega2Euler_dot(omega_b,Euler)

phi = Euler(1);
theta = Euler(2);
psi = Euler(3);


A = [1          0               -sin(theta)         ;
     0          cos(phi)        sin(phi)*cos(theta) ;
     0          -sin(phi)       cos(phi)*cos(theta)];

Euler_dot = A'*omega_b ;

== matlab function dbx_control/Px4_to_simulink input interface/MATLAB Function ==
  data: T_yaw output; yaw input
function T_yaw = Yaw_rotate(yaw)


T_yaw=[cos(yaw),    sin(yaw),   0;
        -sin(yaw),  cos(yaw),   0;
        0,      0,              1];

== matlab function dbx_control/Auto-mode autopiloto/DBX advance control system/Inner PI Controller Euler/MATLAB Function1 ==
  data: Euler_dot input size=[3,1]; Omega output; euler_ang input size=[3,1]
function Omega = Euler_dot_2_omega(Euler_dot,euler_ang)

phi = euler_ang(1);
theta = euler_ang(2);
psi = euler_ang(3);


A = [1          0               -sin(theta)         ;
     0          cos(phi)        sin(phi)*cos(theta) ;
     0          -sin(phi)       cos(phi)*cos(theta)];

Omega = A*Euler_dot ;

== matlab function dbx_control/Auto-mode autopiloto/DBX advance control system/Inner PI Controller Euler/Limits in Ang accel/Limis eval ==
  data: Ang_Accel input size=[3,1]; Limit_up output; Limit_down output; A_M parameter; L_M parameter; m parameter; g parameter; I_BAC parameter
function [Limit_up,Limit_down]= Max_ang_accels(Ang_Accel,A_M,L_M,m,g,I_BAC)

Limit_up=Ang_Accel;
Limit_down=Ang_Accel;

Limit_up(1) =   abs( (2*m*g/3*A_M/2  )/I_BAC(1,1)  )* 0.5 ;
Limit_down(1) = -Limit_up(1) ;

Limit_up(2) = abs(1/3*L_M*m*g*2/3)/I_BAC(2,2)* 0.5 ;
Limit_down(2) = -Limit_up(2);


Limit_up(3) = ( 2/3*L_M*m*g/3*sin(15/180*pi) )/I_BAC(3,3)* 0.5 ;
Limit_down(3) = -Limit_up(3) ;
